simulink model "microgrid_4DER_2019"  (R2019a)
settings: Solver=VariableStepAuto  StartTime=0.0  StopTime=10  RelTol=1e-3
values from neighbouring files (symbols this model uses):
  cf1 = 50 * 1e-6    (= 5e-05)    [parameters.m]
  F1 = 0.75    [parameters.m]
  kic1 = 16e3    (= 16000)    [parameters.m]
  kiv1 = 390    [parameters.m]
  kpc1 = 10.5    [parameters.m]
  kpv1 = 0.05    [parameters.m]
  Lc1 = 0.35 * 1e-3    (= 0.00035)    [parameters.m]
  Lf1 = 1.35 * 1e-3    (= 0.00135)    [parameters.m]
  mp1 = 9.4 * 1e-5    (= 9.4e-05)    [parameters.m]
  nq1 = 1.3 * 1e-3    (= 0.0013)    [parameters.m]
  Rc1 = 0.03    [parameters.m]
  Rf1 = 0.1    [parameters.m]
  Tss = 2.5e-6    (= 2.5e-06)    [parameters.m]
  wb1 = 50 * 2 * pi    (= 314.159265359)    [parameters.m]
  wc1 = 31.41    [parameters.m]
  wcom = 0 * 2 * pi    (= 0)    [parameters.m]
undefined symbols (not defined in the file or in its folder): L11, L12, L13, Lf, R11, R12, R13
libraries: powerlib x46, powerlib_meascontrol x28
(part 1 of 2)
settings Model: Creator=derek  LastModifiedBy=derek

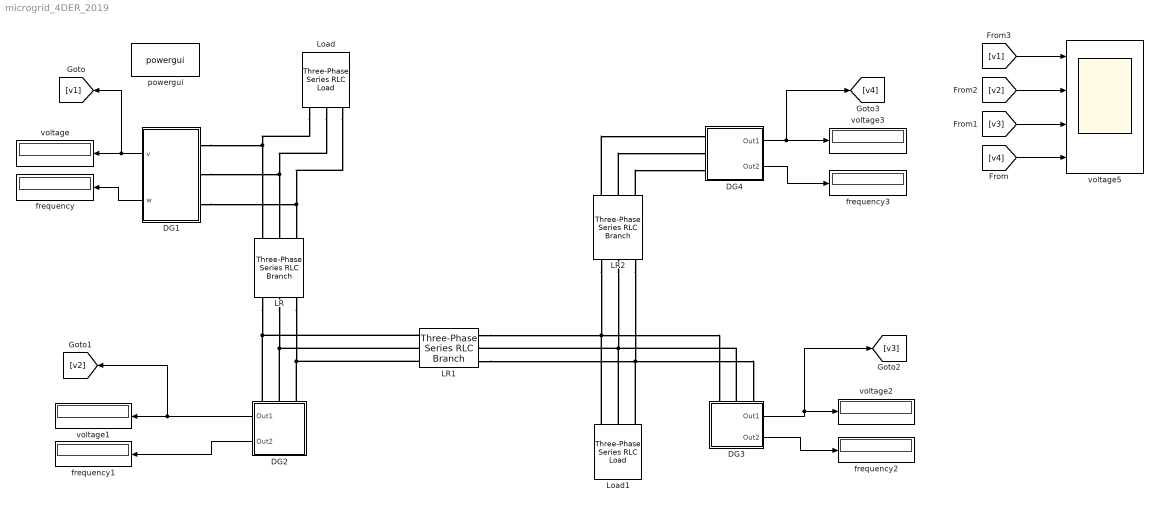
== system microgrid_4DER_2019 ==
  DG1 : Subsystem
  DG2 : Subsystem
      settings: PortSchema="{\"entries\":[{\"content\":{\"sides\":[{\"content\":{\"connectorIds\":[\"LConn1\",\"LConn2\",\"LConn3\"]},\"type\":\"ConnectorPlacement.EquallySpacedRectSide\",\"uuid\":\"9284fba5-743e-4ae1-952f-4876aa99f3ee\"},{\"content\":{\"connectorIds\":[],\"side\":\"RIGHT\"},\"type\":\"ConnectorPlacement.EquallySpacedRectSide\",\"uuid\":\"acb9d5d7-58dc-4066-8a65-0e305600e686\"},{\"content\":{\"connectorIds\":[\"Out1\",\"Out2\"],\"side\":\"TOP\"},\"type\":\"ConnectorPlacement.EquallySpacedRectSide\",\"uuid\":\"239fd259-a6d3-4a4c-98e9-885779a24b56\"}]},\"type\":\"ConnectorPlacement.EquallySpacedConnector\",\"uuid\":\"61a245b7-1af2-4895-a866-301198dca684\"}],\"packageUris\":[\"http://schema.mathworks.com/mf0/Connector/19700101\"],\"version\":\"1.0\"}"
  DG3 : Subsystem
      settings: PortSchema="{\"entries\":[{\"content\":{\"sides\":[{\"content\":{\"connectorIds\":[\"LConn1\",\"LConn2\",\"LConn3\"]},\"type\":\"ConnectorPlacement.EquallySpacedRectSide\",\"uuid\":\"9284fba5-743e-4ae1-952f-4876aa99f3ee\"},{\"content\":{\"connectorIds\":[],\"side\":\"RIGHT\"},\"type\":\"ConnectorPlacement.EquallySpacedRectSide\",\"uuid\":\"acb9d5d7-58dc-4066-8a65-0e305600e686\"},{\"content\":{\"connectorIds\":[],\"side\":\"TOP\"},\"type\":\"ConnectorPlacement.EquallySpacedRectSide\",\"uuid\":\"239fd259-a6d3-4a4c-98e9-885779a24b56\"},{\"content\":{\"connectorIds\":[\"Out1\",\"Out2\"],\"side\":\"BOTTOM\"},\"type\":\"ConnectorPlacement.EquallySpacedRectSide\",\"uuid\":\"f03bd340-3053-4b1f-9b05-34f1428ba472\"}]},\"type\":\"ConnectorPlacement.EquallySpacedConnector\",\"uuid\":\"61a245b7-1af2-4895-a866-301198dca684\"}],\"packageUris\":[\"http://schema.mathworks.com/mf0/Connector/19700101\"],\"version\":\"1.0\"}"
  DG4 : Subsystem
  LR : powerlib/Elements/Three-Phase Series RLC Branch  LConnTagsString=A|B|C  RConnTagsString=A|B|C  BranchType=RL  Resistance=R11  Inductance=L11  Capacitance=Lf  Measurements=None
  LR1 : powerlib/Elements/Three-Phase Series RLC Branch  LConnTagsString=A|B|C  RConnTagsString=A|B|C  BranchType=RL  Resistance=R12  Inductance=L12  Capacitance=Lf  Measurements=None
  LR2 : powerlib/Elements/Three-Phase Series RLC Branch  LConnTagsString=A|B|C  RConnTagsString=A|B|C  BranchType=RL  Resistance=R13  Inductance=L13  Capacitance=Lf  Measurements=None
  Load : powerlib/Elements/Three-Phase Series RLC Load  LConnTagsString=A|B|C  Configuration=Y (grounded)  NominalVoltage=314  Vabc=[1e3 1e3 1e3]  Vabcp=[1e3 1e3 1e3]  NominalFrequency=50  UnbalancedPower=off  ActivePower=12e3  InductivePower=0  CapacitivePower=0  Pabc=[10e3 9e3 11e3]  QLabc=[100 90 110]  QCabc=[100 90 110]  Pabcp=[10e3 9e3 11e3]  QLabcp=[100 90 110]  QCabcp=[100 90 110]  Measurements=None  LoadType=constant Z
  Load1 : powerlib/Elements/Three-Phase Series RLC Load  LConnTagsString=A|B|C  Configuration=Y (grounded)  NominalVoltage=314  Vabc=[1e3 1e3 1e3]  Vabcp=[1e3 1e3 1e3]  NominalFrequency=50  UnbalancedPower=off  ActivePower=15e3  InductivePower=0  CapacitivePower=0  Pabc=[10e3 9e3 11e3]  QLabc=[100 90 110]  QCabc=[100 90 110]  Pabcp=[10e3 9e3 11e3]  QLabcp=[100 90 110]  QCabcp=[100 90 110]  Measurements=None  LoadType=constant Z
  frequency{,1..3} (4 alike) : Display
  powergui : powerlib/powergui  Priority=1  SimulationMode=Discrete  SampleTime=Tss  frequency=60  Iterations=50  frequencyindice=0  Pbase=100e6  ErrMax=1e-4  UnitsV=kV  UnitsW=MW  buscounter=0  FunctionMessages=off  echomessages=off  EnableUseOfTLC=off  CurrentSourceSwitches=off  DisableSnubberDevices=off  DisableRonSwitches=off  DisableVfSwitches=off  DisplayEquations=off  AutomaticDiscreteSolvers=off  SolverType=Tustin/Backward Euler (TBE)  Interpol=off  ExternalGateDelay=off  methode=off  Ts=100  x0status=blocks  SPID=on  SwTol=0  HookPort=off  NonlinearTolerance=0  nMaxIteration=15  ContinueOnMaxIteration=off  RestoreLinks=warning  ResistiveCurrentMeasurement=off  Frange=[0:2:500]  Ylog=off  Xlog=on  ShowGrid=off  save=off  variable=ZData  structure=0  ZoomFFT=off  StartTime=0.0  cycles=1  DisplayStyle=1  fundamental=60  FreqAxis=off  MaxFrequency=1000  frequencyindicesteady=1  RmsSteady=1  display=off
  voltage{,1..3} (4 alike) : Display
  voltage5 : Scope  NumInputPorts=4
  wires:
  DG1/1(v) -> [v1], voltage/1
  DG1/2(w) -> frequency/1
  DG2/1(Out1) -> [v2], voltage1/1
  DG2/2(Out2) -> frequency1/1
  DG4/1(Out1) -> [v4], voltage3/1
  DG4/2(Out2) -> frequency3/1
  DG3/1(Out1) -> [v3], voltage2/1
  DG3/2(Out2) -> frequency2/1
  [v4] -> voltage5/4
  [v3] -> voltage5/3
  [v2] -> voltage5/2
  [v1] -> voltage5/1
  connections:
  DG1/LConn1 -- Load/LConn1 -- LR/LConn1
  DG1/LConn2 -- Load/LConn2 -- LR/LConn2
  DG1/LConn3 -- Load/LConn3 -- LR/LConn3
  LR/RConn1 -- DG2/LConn1 -- LR1/LConn1
  LR/RConn2 -- DG2/LConn2 -- LR1/LConn2
  LR/RConn3 -- DG2/LConn3 -- LR1/LConn3
  LR1/RConn1 -- Load1/LConn1 -- LR2/LConn1 -- DG3/LConn1
  DG3/LConn2 -- LR1/RConn2 -- Load1/LConn2 -- LR2/LConn2
  LR1/RConn3 -- Load1/LConn3 -- LR2/LConn3 -- DG3/LConn3
  LR2/RConn1 -- DG4/LConn1
  LR2/RConn2 -- DG4/LConn2
  LR2/RConn3 -- DG4/LConn3

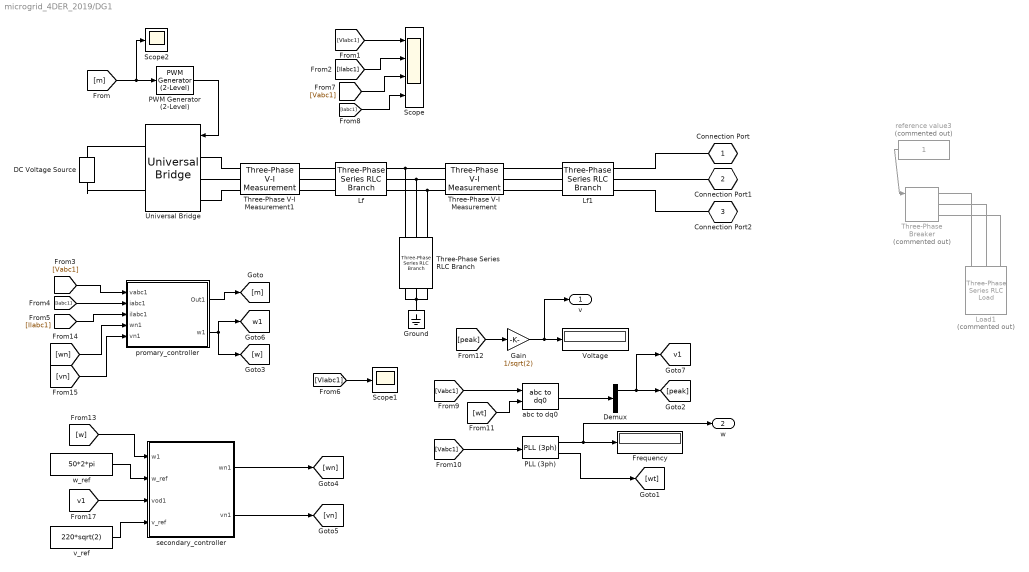
== system microgrid_4DER_2019/DG1 ==
  DC Voltage Source : powerlib/Electrical Sources/DC Voltage Source  Amplitude=600  Measurements=None
  Demux : Demux  Outputs=3
  Frequency : Display
  Gain : Gain  Gain=1/sqrt(2)
  Ground : powerlib/Elements/Ground  LConnTagsString=a
  Lf : powerlib/Elements/Three-Phase Series RLC Branch  LConnTagsString=A|B|C  RConnTagsString=A|B|C  BranchType=RL  Resistance=Rf1  Inductance=Lf1  Capacitance=Lf  Measurements=None
  Lf1 : powerlib/Elements/Three-Phase Series RLC Branch  LConnTagsString=A|B|C  RConnTagsString=A|B|C  BranchType=RL  Resistance=Rc1  Inductance=Lc1  Capacitance=Lf  Measurements=None
  Load1 : powerlib/Elements/Three-Phase Series RLC Load  Commented=on  LConnTagsString=A|B|C  Configuration=Y (grounded)  NominalVoltage=314  Vabc=[1e3 1e3 1e3]  Vabcp=[1e3 1e3 1e3]  NominalFrequency=50  UnbalancedPower=off  ActivePower=20e3  InductivePower=0  CapacitivePower=0  Pabc=[10e3 9e3 11e3]  QLabc=[100 90 110]  QCabc=[100 90 110]  Pabcp=[10e3 9e3 11e3]  QLabcp=[100 90 110]  QCabcp=[100 90 110]  Measurements=None  LoadType=constant Z
  PLL (3ph) : powerlib_meascontrol/PLL/PLL (3ph)  Fmin=45  Par_Init=[0, 50]  ParK=[180, 3200, 1]  TcD=1e-4  MaxRateChangeFreq=12  FilterCutOffFreq=25  Ts=Tss  AGC=on
  PWM Generator (2-Level) : powerlib_meascontrol/Pulse & Signal Generators/PWM Generator (2-Level)  ModulatorType=Three-phase bridge (6 pulses)  ModulatorMode=Unsynchronized  Fc=fsw  Pc=90  nF=27  MinMax="[ -1  1 ]"  SamplingTechnique=Natural  ModulatingSignals=off  m=0.8  Freq=60  Phase=0  Ts=Tss  ShowCarrierOutport=off
  Scope : Scope  NumInputPorts=4
  Scope1 : Scope
  Scope2 : Scope
  Three-Phase Series RLC Branch : powerlib/Elements/Three-Phase Series RLC Branch  LConnTagsString=A|B|C  RConnTagsString=A|B|C  BranchType=RC  Resistance=1e-6  Inductance=1e-3  Capacitance=cf1  Measurements=None
  Three-Phase V-I Measurement : powerlib/Measurements/Three-Phase V-I Measurement  VoltageMeasurement=phase-to-phase  SetLabelV=on  LabelV=Vabc1  Vpu=off  VpuLL=off  CurrentMeasurement=yes  SetLabelI=on  LabelI=Iabc1  Ipu=off  Pbase=100e6  Vbase=500e3  OutputType=Complex  PhasorSimulation=off  PSBequivalent=0
  Three-Phase V-I Measurement1 : powerlib/Measurements/Three-Phase V-I Measurement  VoltageMeasurement=phase-to-phase  SetLabelV=on  LabelV=Vlabc1  Vpu=off  VpuLL=off  CurrentMeasurement=yes  SetLabelI=on  LabelI=Ilabc1  Ipu=off  Pbase=100e6  Vbase=500e3  OutputType=Complex  PhasorSimulation=off  PSBequivalent=0
  Three-Phase Breaker : powerlib/Elements/Three-Phase Breaker  Commented=on  InitialState=open  SwitchA=on  SwitchB=on  SwitchC=on  SwitchTimes="[1/60  5/60]"  External=on  BreakerResistance=0.01  SnubberResistance=1e6  SnubberCapacitance=inf  Measurements=None
  Universal Bridge : powerlib/Power Electronics/Universal Bridge  Arms=3  SnubberResistance=1e5  SnubberCapacitance=inf  Device=IGBT / Diodes  Ron=1e-3  Lon=0  ForwardVoltages="[  0  0  ]"  ForwardVoltage=0  GTOparameters=[ 10e-6 , 20e-6 ]  IGBTparameters=[ 1e-6 , 2e-6 ]  Measurements=None  Measurements_2=None  converterType=Rectifier
  Voltage : Display
  abc to dq0 : powerlib_meascontrol/Transformations/abc to dq0  Alignment=90 degrees behind phase A axis
  promary_controller : Subsystem
  reference value3 : Constant  Commented=on
  secondary_controller : Subsystem
  v_ref : Constant  Value=220*sqrt(2)
  w_ref : Constant  Value=50*2*pi
  Connection Port : PMIOPort  Tag=PMCPort  Side=Left
  Connection Port1 : PMIOPort  Tag=PMCPort  Port=2  Side=Left
  Connection Port2 : PMIOPort  Tag=PMCPort  Port=3  Side=Left
  v : Outport
  w : Outport  Port=2
  tag scope: v1=global, w1=global
  wires:
  [Ilabc1] -> Scope/2
  [Iabc1] -> Scope/4
  [Iabc1] -> promary_controller/2(iabc1)
  [Vlabc1] -> Scope1/1
  [Vlabc1] -> Scope/1
  Gain/1 -> v/1, Voltage/1
  PLL (3ph)/2 -> [wt]
  reference value3/1 -> Three-Phase Breaker/1
  PWM Generator (2-Level)/1 -> Universal Bridge/1
  [Ilabc1] -> promary_controller/3(ilabc1)
  [Vabc1] -> promary_controller/1(vabc1)
  Demux/1 -> [v1], [peak]
  abc to dq0/1 -> Demux/1
  [Vabc1] -> abc to dq0/1
  [Vabc1] -> PLL (3ph)/1
  promary_controller/1(Out1) -> [m]
  [peak] -> Gain/1
  [wt] -> abc to dq0/2
  [m] -> Scope2/1, PWM Generator (2-Level)/1
  PLL (3ph)/1 -> w/1, Frequency/1
  [Vabc1] -> Scope/3
  [w] -> secondary_controller/1(w1)
  promary_controller/2(w1) -> [w1], [w]
  v_ref/1 -> secondary_controller/4(v_ref)
  secondary_controller/1(wn1) -> [wn]
  [wn] -> promary_controller/4(wn1)
  secondary_controller/2(vn1) -> [vn]
  [vn] -> promary_controller/5(vn1)
  [v1] -> secondary_controller/3(vod1)
  w_ref/1 -> secondary_controller/2(w_ref)
  connections:
  Lf1/LConn3 -- Three-Phase V-I Measurement/RConn3
  Three-Phase Breaker/RConn2 -- Load1/LConn2
  Lf1/LConn2 -- Three-Phase V-I Measurement/RConn2
  Connection Port2/RConn1 -- Lf1/RConn3
  Three-Phase Breaker/RConn3 -- Load1/LConn3
  Three-Phase V-I Measurement1/RConn3 -- Lf/LConn3
  Three-Phase V-I Measurement/RConn1 -- Lf1/LConn1
  Three-Phase V-I Measurement1/LConn3 -- Universal Bridge/LConn3
  Three-Phase V-I Measurement1/RConn2 -- Lf/LConn2
  Ground/LConn1 -- Three-Phase Series RLC Branch/RConn3 -- Three-Phase Series RLC Branch/RConn2 -- Three-Phase Series RLC Branch/RConn1
  Lf/RConn2 -- Three-Phase V-I Measurement/LConn2 -- Three-Phase Series RLC Branch/LConn2
  Three-Phase V-I Measurement1/RConn1 -- Lf/LConn1
  Three-Phase V-I Measurement1/LConn2 -- Universal Bridge/LConn2
  Connection Port/RConn1 -- Lf1/RConn1
  DC Voltage Source/RConn1 -- Universal Bridge/RConn1
  Connection Port1/RConn1 -- Lf1/RConn2
  Lf/RConn3 -- Three-Phase V-I Measurement/LConn3 -- Three-Phase Series RLC Branch/LConn3
  Three-Phase Breaker/RConn1 -- Load1/LConn1
  Lf/RConn1 -- Three-Phase V-I Measurement/LConn1 -- Three-Phase Series RLC Branch/LConn1
  DC Voltage Source/LConn1 -- Universal Bridge/RConn2
  Universal Bridge/LConn1 -- Three-Phase V-I Measurement1/LConn1

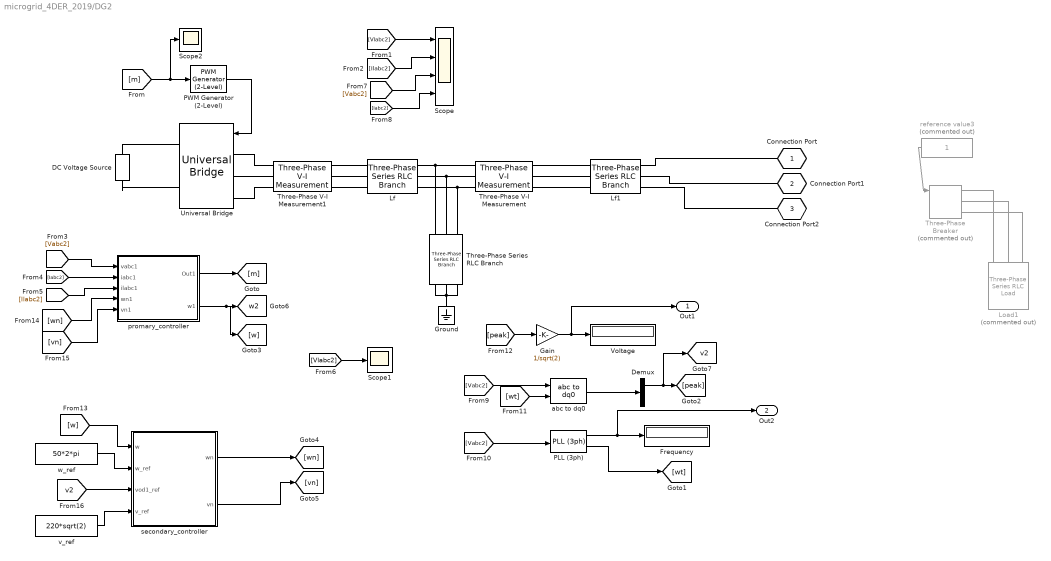
== system microgrid_4DER_2019/DG2 ==
  DC Voltage Source : powerlib/Electrical Sources/DC Voltage Source  Amplitude=600  Measurements=None
  Demux : Demux  Outputs=3
  Frequency : Display
  Gain : Gain  Gain=1/sqrt(2)
  Ground : powerlib/Elements/Ground  LConnTagsString=a
  Lf : powerlib/Elements/Three-Phase Series RLC Branch  LConnTagsString=A|B|C  RConnTagsString=A|B|C  BranchType=RL  Resistance=Rf1  Inductance=Lf1  Capacitance=Lf  Measurements=None
  Lf1 : powerlib/Elements/Three-Phase Series RLC Branch  LConnTagsString=A|B|C  RConnTagsString=A|B|C  BranchType=RL  Resistance=Rc1  Inductance=Lc1  Capacitance=Lf  Measurements=None
  Load1 : powerlib/Elements/Three-Phase Series RLC Load  Commented=on  LConnTagsString=A|B|C  Configuration=Y (grounded)  NominalVoltage=314  Vabc=[1e3 1e3 1e3]  Vabcp=[1e3 1e3 1e3]  NominalFrequency=50  UnbalancedPower=off  ActivePower=20e3  InductivePower=0  CapacitivePower=0  Pabc=[10e3 9e3 11e3]  QLabc=[100 90 110]  QCabc=[100 90 110]  Pabcp=[10e3 9e3 11e3]  QLabcp=[100 90 110]  QCabcp=[100 90 110]  Measurements=None  LoadType=constant Z
  PLL (3ph) : powerlib_meascontrol/PLL/PLL (3ph)  Fmin=45  Par_Init=[0, 50]  ParK=[180, 3200, 1]  TcD=1e-4  MaxRateChangeFreq=12  FilterCutOffFreq=25  Ts=Tss  AGC=on
  PWM Generator (2-Level) : powerlib_meascontrol/Pulse & Signal Generators/PWM Generator (2-Level)  ModulatorType=Three-phase bridge (6 pulses)  ModulatorMode=Unsynchronized  Fc=fsw  Pc=90  nF=27  MinMax="[ -1  1 ]"  SamplingTechnique=Natural  ModulatingSignals=off  m=0.8  Freq=60  Phase=0  Ts=Tss  ShowCarrierOutport=off
  Scope : Scope  NumInputPorts=4
  Scope1 : Scope
  Scope2 : Scope
  Three-Phase Series RLC Branch : powerlib/Elements/Three-Phase Series RLC Branch  LConnTagsString=A|B|C  RConnTagsString=A|B|C  BranchType=RC  Resistance=1e-6  Inductance=1e-3  Capacitance=cf1  Measurements=None
  Three-Phase V-I Measurement : powerlib/Measurements/Three-Phase V-I Measurement  VoltageMeasurement=phase-to-phase  SetLabelV=on  LabelV=Vabc2  Vpu=off  VpuLL=off  CurrentMeasurement=yes  SetLabelI=on  LabelI=Iabc2  Ipu=off  Pbase=100e6  Vbase=500e3  OutputType=Complex  PhasorSimulation=off  PSBequivalent=0
  Three-Phase V-I Measurement1 : powerlib/Measurements/Three-Phase V-I Measurement  VoltageMeasurement=phase-to-phase  SetLabelV=on  LabelV=Vlabc2  Vpu=off  VpuLL=off  CurrentMeasurement=yes  SetLabelI=on  LabelI=Ilabc2  Ipu=off  Pbase=100e6  Vbase=500e3  OutputType=Complex  PhasorSimulation=off  PSBequivalent=0
  Three-Phase Breaker : powerlib/Elements/Three-Phase Breaker  Commented=on  InitialState=open  SwitchA=on  SwitchB=on  SwitchC=on  SwitchTimes="[1/60  5/60]"  External=on  BreakerResistance=0.01  SnubberResistance=1e6  SnubberCapacitance=inf  Measurements=None
  Universal Bridge : powerlib/Power Electronics/Universal Bridge  Arms=3  SnubberResistance=1e5  SnubberCapacitance=inf  Device=IGBT / Diodes  Ron=1e-3  Lon=0  ForwardVoltages="[  0  0  ]"  ForwardVoltage=0  GTOparameters=[ 10e-6 , 20e-6 ]  IGBTparameters=[ 1e-6 , 2e-6 ]  Measurements=None  Measurements_2=None  converterType=Rectifier
  Voltage : Display
  abc to dq0 : powerlib_meascontrol/Transformations/abc to dq0  Alignment=90 degrees behind phase A axis
  promary_controller : Subsystem
  reference value3 : Constant  Commented=on
  secondary_controller : Subsystem
  v_ref : Constant  Value=220*sqrt(2)
  w_ref : Constant  Value=50*2*pi
  Connection Port : PMIOPort  Tag=PMCPort  Side=Left
  Connection Port1 : PMIOPort  Tag=PMCPort  Port=2  Side=Left
  Connection Port2 : PMIOPort  Tag=PMCPort  Port=3  Side=Left
  Out1 : Outport
  Out2 : Outport  Port=2
  tag scope: v2=global, w2=global
  wires:
  [Ilabc2] -> Scope/2
  [Iabc2] -> Scope/4
  [Vlabc2] -> Scope1/1
  [Vlabc2] -> Scope/1
  Gain/1 -> Out1/1, Voltage/1
  PLL (3ph)/2 -> [wt]
  reference value3/1 -> Three-Phase Breaker/1
  PWM Generator (2-Level)/1 -> Universal Bridge/1
  Demux/1 -> [v2], [peak]
  abc to dq0/1 -> Demux/1
  [Vabc2] -> abc to dq0/1
  [Vabc2] -> PLL (3ph)/1
  [peak] -> Gain/1
  [wt] -> abc to dq0/2
  [m] -> Scope2/1, PWM Generator (2-Level)/1
  PLL (3ph)/1 -> Out2/1, Frequency/1
  [Vabc2] -> Scope/3
  [Iabc2] -> promary_controller/2(iabc1)
  [Vabc2] -> promary_controller/1(vabc1)
  [wn] -> promary_controller/4(wn1)
  promary_controller/1(Out1) -> [m]
  promary_controller/2(w1) -> [w], [w2]
  [vn] -> promary_controller/5(vn1)
  [Ilabc2] -> promary_controller/3(ilabc1)
  secondary_controller/2(vn) -> [vn]
  secondary_controller/1(wn) -> [wn]
  [v2] -> secondary_controller/3(vod1_ref)
  w_ref/1 -> secondary_controller/2(w_ref)
  [w] -> secondary_controller/1(w)
  v_ref/1 -> secondary_controller/4(v_ref)
  connections:
  Lf1/LConn3 -- Three-Phase V-I Measurement/RConn3
  Three-Phase Breaker/RConn2 -- Load1/LConn2
  Lf1/LConn2 -- Three-Phase V-I Measurement/RConn2
  Connection Port2/RConn1 -- Lf1/RConn3
  Three-Phase Breaker/RConn3 -- Load1/LConn3
  Three-Phase V-I Measurement1/RConn3 -- Lf/LConn3
  Three-Phase V-I Measurement/RConn1 -- Lf1/LConn1
  Three-Phase V-I Measurement1/LConn3 -- Universal Bridge/LConn3
  Three-Phase V-I Measurement1/RConn2 -- Lf/LConn2
  Ground/LConn1 -- Three-Phase Series RLC Branch/RConn3 -- Three-Phase Series RLC Branch/RConn2 -- Three-Phase Series RLC Branch/RConn1
  Lf/RConn2 -- Three-Phase V-I Measurement/LConn2 -- Three-Phase Series RLC Branch/LConn2
  Three-Phase V-I Measurement1/RConn1 -- Lf/LConn1
  Three-Phase V-I Measurement1/LConn2 -- Universal Bridge/LConn2
  Connection Port/RConn1 -- Lf1/RConn1
  DC Voltage Source/RConn1 -- Universal Bridge/RConn1
  Connection Port1/RConn1 -- Lf1/RConn2
  Lf/RConn3 -- Three-Phase V-I Measurement/LConn3 -- Three-Phase Series RLC Branch/LConn3
  Three-Phase Breaker/RConn1 -- Load1/LConn1
  Lf/RConn1 -- Three-Phase V-I Measurement/LConn1 -- Three-Phase Series RLC Branch/LConn1
  DC Voltage Source/LConn1 -- Universal Bridge/RConn2
  Universal Bridge/LConn1 -- Three-Phase V-I Measurement1/LConn1

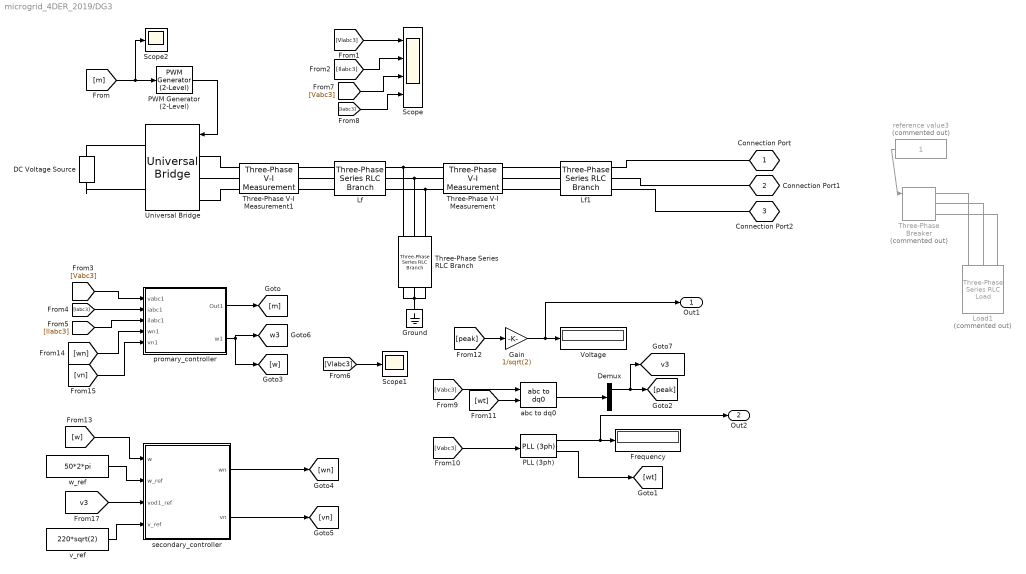
== system microgrid_4DER_2019/DG3 ==
  DC Voltage Source : powerlib/Electrical Sources/DC Voltage Source  Amplitude=600  Measurements=None
  Demux : Demux  Outputs=3
  Frequency : Display
  Gain : Gain  Gain=1/sqrt(2)
  Ground : powerlib/Elements/Ground  LConnTagsString=a
  Lf : powerlib/Elements/Three-Phase Series RLC Branch  LConnTagsString=A|B|C  RConnTagsString=A|B|C  BranchType=RL  Resistance=Rf1  Inductance=Lf1  Capacitance=Lf  Measurements=None
  Lf1 : powerlib/Elements/Three-Phase Series RLC Branch  LConnTagsString=A|B|C  RConnTagsString=A|B|C  BranchType=RL  Resistance=Rc1  Inductance=Lc1  Capacitance=Lf  Measurements=None
  Load1 : powerlib/Elements/Three-Phase Series RLC Load  Commented=on  LConnTagsString=A|B|C  Configuration=Y (grounded)  NominalVoltage=314  Vabc=[1e3 1e3 1e3]  Vabcp=[1e3 1e3 1e3]  NominalFrequency=50  UnbalancedPower=off  ActivePower=20e3  InductivePower=0  CapacitivePower=0  Pabc=[10e3 9e3 11e3]  QLabc=[100 90 110]  QCabc=[100 90 110]  Pabcp=[10e3 9e3 11e3]  QLabcp=[100 90 110]  QCabcp=[100 90 110]  Measurements=None  LoadType=constant Z
  PLL (3ph) : powerlib_meascontrol/PLL/PLL (3ph)  Fmin=45  Par_Init=[0, 50]  ParK=[180, 3200, 1]  TcD=1e-4  MaxRateChangeFreq=12  FilterCutOffFreq=25  Ts=Tss  AGC=on
  PWM Generator (2-Level) : powerlib_meascontrol/Pulse & Signal Generators/PWM Generator (2-Level)  ModulatorType=Three-phase bridge (6 pulses)  ModulatorMode=Unsynchronized  Fc=fsw  Pc=90  nF=27  MinMax="[ -1  1 ]"  SamplingTechnique=Natural  ModulatingSignals=off  m=0.8  Freq=60  Phase=0  Ts=Tss  ShowCarrierOutport=off
  Scope : Scope  NumInputPorts=4
  Scope1 : Scope
  Scope2 : Scope
  Three-Phase Series RLC Branch : powerlib/Elements/Three-Phase Series RLC Branch  LConnTagsString=A|B|C  RConnTagsString=A|B|C  BranchType=RC  Resistance=1e-6  Inductance=1e-3  Capacitance=cf1  Measurements=None
  Three-Phase V-I Measurement : powerlib/Measurements/Three-Phase V-I Measurement  VoltageMeasurement=phase-to-phase  SetLabelV=on  LabelV=Vabc3  Vpu=off  VpuLL=off  CurrentMeasurement=yes  SetLabelI=on  LabelI=Iabc3  Ipu=off  Pbase=100e6  Vbase=500e3  OutputType=Complex  PhasorSimulation=off  PSBequivalent=0
  Three-Phase V-I Measurement1 : powerlib/Measurements/Three-Phase V-I Measurement  VoltageMeasurement=phase-to-phase  SetLabelV=on  LabelV=Vlabc3  Vpu=off  VpuLL=off  CurrentMeasurement=yes  SetLabelI=on  LabelI=Ilabc3  Ipu=off  Pbase=100e6  Vbase=500e3  OutputType=Complex  PhasorSimulation=off  PSBequivalent=0
  Three-Phase Breaker : powerlib/Elements/Three-Phase Breaker  Commented=on  InitialState=open  SwitchA=on  SwitchB=on  SwitchC=on  SwitchTimes="[1/60  5/60]"  External=on  BreakerResistance=0.01  SnubberResistance=1e6  SnubberCapacitance=inf  Measurements=None
  Universal Bridge : powerlib/Power Electronics/Universal Bridge  Arms=3  SnubberResistance=1e5  SnubberCapacitance=inf  Device=IGBT / Diodes  Ron=1e-3  Lon=0  ForwardVoltages="[  0  0  ]"  ForwardVoltage=0  GTOparameters=[ 10e-6 , 20e-6 ]  IGBTparameters=[ 1e-6 , 2e-6 ]  Measurements=None  Measurements_2=None  converterType=Rectifier
  Voltage : Display
  abc to dq0 : powerlib_meascontrol/Transformations/abc to dq0  Alignment=90 degrees behind phase A axis
  promary_controller : Subsystem
  reference value3 : Constant  Commented=on
  secondary_controller : Subsystem
  v_ref : Constant  Value=220*sqrt(2)
  w_ref : Constant  Value=50*2*pi
  Connection Port : PMIOPort  Tag=PMCPort  Side=Left
  Connection Port1 : PMIOPort  Tag=PMCPort  Port=2  Side=Left
  Connection Port2 : PMIOPort  Tag=PMCPort  Port=3  Side=Left
  Out1 : Outport
  Out2 : Outport  Port=2
  tag scope: v3=global, w3=global
  wires:
  [Ilabc3] -> Scope/2
  [Iabc3] -> Scope/4
  [Vlabc3] -> Scope1/1
  [Vlabc3] -> Scope/1
  Gain/1 -> Out1/1, Voltage/1
  PLL (3ph)/2 -> [wt]
  reference value3/1 -> Three-Phase Breaker/1
  PWM Generator (2-Level)/1 -> Universal Bridge/1
  Demux/1 -> [peak], [v3]
  abc to dq0/1 -> Demux/1
  [Vabc3] -> abc to dq0/1
  [Vabc3] -> PLL (3ph)/1
  [peak] -> Gain/1
  [wt] -> abc to dq0/2
  [m] -> Scope2/1, PWM Generator (2-Level)/1
  PLL (3ph)/1 -> Out2/1, Frequency/1
  [Vabc3] -> Scope/3
  [Vabc3] -> promary_controller/1(vabc1)
  [Ilabc3] -> promary_controller/3(ilabc1)
  [wn] -> promary_controller/4(wn1)
  promary_controller/2(w1) -> [w3], [w]
  [Iabc3] -> promary_controller/2(iabc1)
  [vn] -> promary_controller/5(vn1)
  promary_controller/1(Out1) -> [m]
  [v3] -> secondary_controller/3(vod1_ref)
  [w] -> secondary_controller/1(w)
  v_ref/1 -> secondary_controller/4(v_ref)
  w_ref/1 -> secondary_controller/2(w_ref)
  secondary_controller/1(wn) -> [wn]
  secondary_controller/2(vn) -> [vn]
  connections:
  Lf1/LConn3 -- Three-Phase V-I Measurement/RConn3
  Three-Phase Breaker/RConn2 -- Load1/LConn2
  Lf1/LConn2 -- Three-Phase V-I Measurement/RConn2
  Connection Port2/RConn1 -- Lf1/RConn3
  Three-Phase Breaker/RConn3 -- Load1/LConn3
  Three-Phase V-I Measurement1/RConn3 -- Lf/LConn3
  Three-Phase V-I Measurement/RConn1 -- Lf1/LConn1
  Three-Phase V-I Measurement1/LConn3 -- Universal Bridge/LConn3
  Three-Phase V-I Measurement1/RConn2 -- Lf/LConn2
  Ground/LConn1 -- Three-Phase Series RLC Branch/RConn3 -- Three-Phase Series RLC Branch/RConn2 -- Three-Phase Series RLC Branch/RConn1
  Lf/RConn2 -- Three-Phase V-I Measurement/LConn2 -- Three-Phase Series RLC Branch/LConn2
  Three-Phase V-I Measurement1/RConn1 -- Lf/LConn1
  Three-Phase V-I Measurement1/LConn2 -- Universal Bridge/LConn2
  Connection Port/RConn1 -- Lf1/RConn1
  DC Voltage Source/RConn1 -- Universal Bridge/RConn1
  Connection Port1/RConn1 -- Lf1/RConn2
  Lf/RConn3 -- Three-Phase V-I Measurement/LConn3 -- Three-Phase Series RLC Branch/LConn3
  Three-Phase Breaker/RConn1 -- Load1/LConn1
  Lf/RConn1 -- Three-Phase V-I Measurement/LConn1 -- Three-Phase Series RLC Branch/LConn1
  DC Voltage Source/LConn1 -- Universal Bridge/RConn2
  Universal Bridge/LConn1 -- Three-Phase V-I Measurement1/LConn1

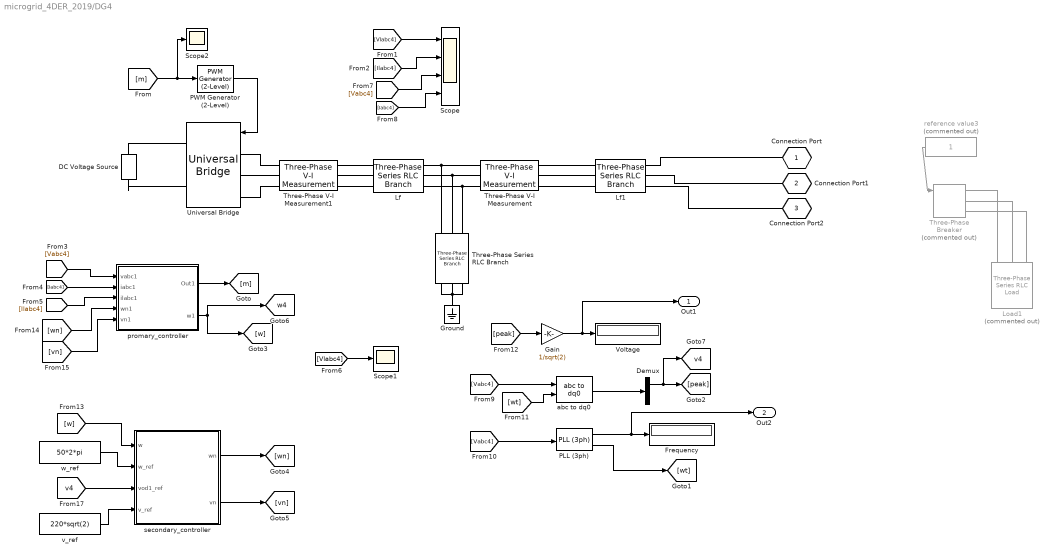
== system microgrid_4DER_2019/DG4 ==
  DC Voltage Source : powerlib/Electrical Sources/DC Voltage Source  Amplitude=600  Measurements=None
  Demux : Demux  Outputs=3
  Frequency : Display
  Gain : Gain  Gain=1/sqrt(2)
  Ground : powerlib/Elements/Ground  LConnTagsString=a
  Lf : powerlib/Elements/Three-Phase Series RLC Branch  LConnTagsString=A|B|C  RConnTagsString=A|B|C  BranchType=RL  Resistance=Rf1  Inductance=Lf1  Capacitance=Lf  Measurements=None
  Lf1 : powerlib/Elements/Three-Phase Series RLC Branch  LConnTagsString=A|B|C  RConnTagsString=A|B|C  BranchType=RL  Resistance=Rc1  Inductance=Lc1  Capacitance=Lf  Measurements=None
  Load1 : powerlib/Elements/Three-Phase Series RLC Load  Commented=on  LConnTagsString=A|B|C  Configuration=Y (grounded)  NominalVoltage=314  Vabc=[1e3 1e3 1e3]  Vabcp=[1e3 1e3 1e3]  NominalFrequency=50  UnbalancedPower=off  ActivePower=20e3  InductivePower=0  CapacitivePower=0  Pabc=[10e3 9e3 11e3]  QLabc=[100 90 110]  QCabc=[100 90 110]  Pabcp=[10e3 9e3 11e3]  QLabcp=[100 90 110]  QCabcp=[100 90 110]  Measurements=None  LoadType=constant Z
  PLL (3ph) : powerlib_meascontrol/PLL/PLL (3ph)  Fmin=45  Par_Init=[0, 50]  ParK=[180, 3200, 1]  TcD=1e-4  MaxRateChangeFreq=12  FilterCutOffFreq=25  Ts=Tss  AGC=on
  PWM Generator (2-Level) : powerlib_meascontrol/Pulse & Signal Generators/PWM Generator (2-Level)  ModulatorType=Three-phase bridge (6 pulses)  ModulatorMode=Unsynchronized  Fc=fsw  Pc=90  nF=27  MinMax="[ -1  1 ]"  SamplingTechnique=Natural  ModulatingSignals=off  m=0.8  Freq=60  Phase=0  Ts=Tss  ShowCarrierOutport=off
  Scope : Scope  NumInputPorts=4
  Scope1 : Scope
  Scope2 : Scope
  Three-Phase Series RLC Branch : powerlib/Elements/Three-Phase Series RLC Branch  LConnTagsString=A|B|C  RConnTagsString=A|B|C  BranchType=RC  Resistance=1e-6  Inductance=1e-3  Capacitance=cf1  Measurements=None
  Three-Phase V-I Measurement : powerlib/Measurements/Three-Phase V-I Measurement  VoltageMeasurement=phase-to-phase  SetLabelV=on  LabelV=Vabc4  Vpu=off  VpuLL=off  CurrentMeasurement=yes  SetLabelI=on  LabelI=Iabc4  Ipu=off  Pbase=100e6  Vbase=500e3  OutputType=Complex  PhasorSimulation=off  PSBequivalent=0
  Three-Phase V-I Measurement1 : powerlib/Measurements/Three-Phase V-I Measurement  VoltageMeasurement=phase-to-phase  SetLabelV=on  LabelV=Vlabc4  Vpu=off  VpuLL=off  CurrentMeasurement=yes  SetLabelI=on  LabelI=Ilabc4  Ipu=off  Pbase=100e6  Vbase=500e3  OutputType=Complex  PhasorSimulation=off  PSBequivalent=0
  Three-Phase Breaker : powerlib/Elements/Three-Phase Breaker  Commented=on  InitialState=open  SwitchA=on  SwitchB=on  SwitchC=on  SwitchTimes="[1/60  5/60]"  External=on  BreakerResistance=0.01  SnubberResistance=1e6  SnubberCapacitance=inf  Measurements=None
  Universal Bridge : powerlib/Power Electronics/Universal Bridge  Arms=3  SnubberResistance=1e5  SnubberCapacitance=inf  Device=IGBT / Diodes  Ron=1e-3  Lon=0  ForwardVoltages="[  0  0  ]"  ForwardVoltage=0  GTOparameters=[ 10e-6 , 20e-6 ]  IGBTparameters=[ 1e-6 , 2e-6 ]  Measurements=None  Measurements_2=None  converterType=Rectifier
  Voltage : Display
  abc to dq0 : powerlib_meascontrol/Transformations/abc to dq0  Alignment=90 degrees behind phase A axis
  promary_controller : Subsystem
  reference value3 : Constant  Commented=on
  secondary_controller : Subsystem
  v_ref : Constant  Value=220*sqrt(2)
  w_ref : Constant  Value=50*2*pi
  Connection Port : PMIOPort  Tag=PMCPort  Side=Left
  Connection Port1 : PMIOPort  Tag=PMCPort  Port=2  Side=Left
  Connection Port2 : PMIOPort  Tag=PMCPort  Port=3  Side=Left
  Out1 : Outport
  Out2 : Outport  Port=2
  tag scope: v4=global, w4=global
  wires:
  [Ilabc4] -> Scope/2
  [Iabc4] -> Scope/4
  [Vlabc4] -> Scope1/1
  [Vlabc4] -> Scope/1
  Gain/1 -> Out1/1, Voltage/1
  PLL (3ph)/2 -> [wt]
  reference value3/1 -> Three-Phase Breaker/1
  PWM Generator (2-Level)/1 -> Universal Bridge/1
  Demux/1 -> [v4], [peak]
  abc to dq0/1 -> Demux/1
  [Vabc4] -> abc to dq0/1
  [Vabc4] -> PLL (3ph)/1
  [peak] -> Gain/1
  [wt] -> abc to dq0/2
  [m] -> Scope2/1, PWM Generator (2-Level)/1
  PLL (3ph)/1 -> Out2/1, Frequency/1
  [Vabc4] -> Scope/3
  [Vabc4] -> promary_controller/1(vabc1)
  [Ilabc4] -> promary_controller/3(ilabc1)
  [wn] -> promary_controller/4(wn1)
  promary_controller/2(w1) -> [w4], [w]
  [Iabc4] -> promary_controller/2(iabc1)
  [vn] -> promary_controller/5(vn1)
  promary_controller/1(Out1) -> [m]
  w_ref/1 -> secondary_controller/2(w_ref)
  v_ref/1 -> secondary_controller/4(v_ref)
  secondary_controller/1(wn) -> [wn]
  secondary_controller/2(vn) -> [vn]
  [w] -> secondary_controller/1(w)
  [v4] -> secondary_controller/3(vod1_ref)
  connections:
  Lf1/LConn3 -- Three-Phase V-I Measurement/RConn3
  Three-Phase Breaker/RConn2 -- Load1/LConn2
  Lf1/LConn2 -- Three-Phase V-I Measurement/RConn2
  Connection Port2/RConn1 -- Lf1/RConn3
  Three-Phase Breaker/RConn3 -- Load1/LConn3
  Three-Phase V-I Measurement1/RConn3 -- Lf/LConn3
  Three-Phase V-I Measurement/RConn1 -- Lf1/LConn1
  Three-Phase V-I Measurement1/LConn3 -- Universal Bridge/LConn3
  Three-Phase V-I Measurement1/RConn2 -- Lf/LConn2
  Ground/LConn1 -- Three-Phase Series RLC Branch/RConn3 -- Three-Phase Series RLC Branch/RConn2 -- Three-Phase Series RLC Branch/RConn1
  Lf/RConn2 -- Three-Phase V-I Measurement/LConn2 -- Three-Phase Series RLC Branch/LConn2
  Three-Phase V-I Measurement1/RConn1 -- Lf/LConn1
  Three-Phase V-I Measurement1/LConn2 -- Universal Bridge/LConn2
  Connection Port/RConn1 -- Lf1/RConn1
  DC Voltage Source/RConn1 -- Universal Bridge/RConn1
  Connection Port1/RConn1 -- Lf1/RConn2
  Lf/RConn3 -- Three-Phase V-I Measurement/LConn3 -- Three-Phase Series RLC Branch/LConn3
  Three-Phase Breaker/RConn1 -- Load1/LConn1
  Lf/RConn1 -- Three-Phase V-I Measurement/LConn1 -- Three-Phase Series RLC Branch/LConn1
  DC Voltage Source/LConn1 -- Universal Bridge/RConn2
  Universal Bridge/LConn1 -- Three-Phase V-I Measurement1/LConn1

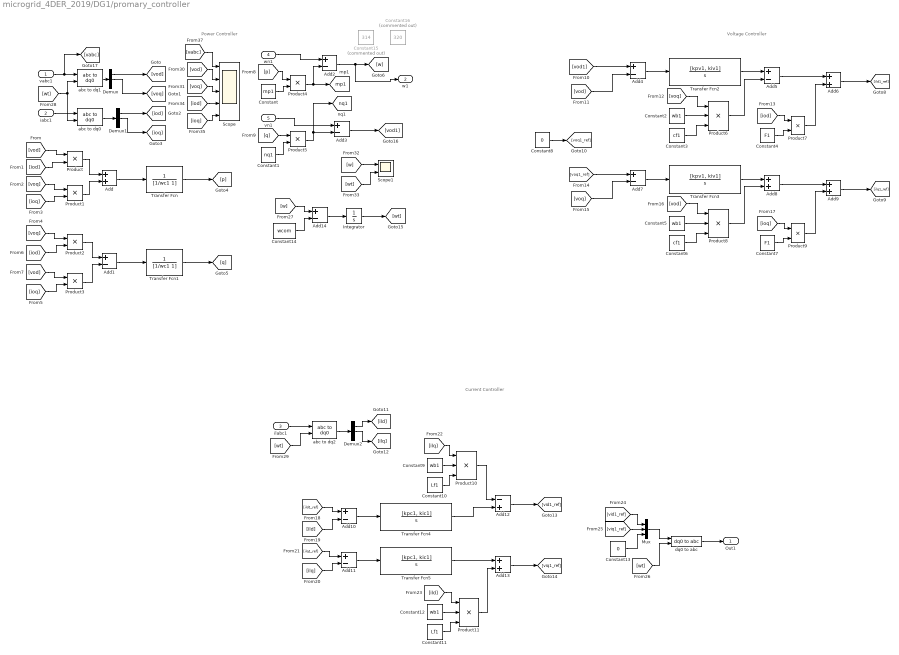
== system microgrid_4DER_2019/DG1/promary_controller ==
  note: Voltage Controller
  note: Power Controller
  note: Current Controller
  vabc1 : Inport
  iabc1 : Inport  Port=2
  ilabc1 : Inport  Port=3
  wn1 : Inport  Port=4
  vn1 : Inport  Port=5
  Add{,6,8..9,13} (5 alike) : Sum
  Add{1..5,7,10..11,14} (9 alike) : Sum  Inputs=+-
  Add12 : Sum  Inputs=-+
  Constant : Constant  Value=mp1
  Constant1 : Constant  Value=nq1
  Constant10 : Constant  Value=Lf1
  Constant11 : Constant  Value=Lf1
  Constant{2,5,9,12} (4 alike) : Constant  Value=wb1
  Constant13 : Constant  Value=0
  Constant14 : Constant  Value=wcom  SampleTime=Tss
  Constant15 : Constant  Commented=on  Value=314
  Constant16 : Constant  Commented=on  Value=320
  Constant3 : Constant  Value=cf1
  Constant4 : Constant  Value=F1
  Constant6 : Constant  Value=cf1
  Constant7 : Constant  Value=F1
  Constant8 : Constant  Value=0
  Demux : Demux  Outputs=3
  Demux1 : Demux  Outputs=3
  Demux2 : Demux  Outputs=3
  Integrator : Integrator
  Mux : Mux  Inputs=3
  Product{,1..5,7,9} (8 alike) : Product
  Product{6,8,10..11} (4 alike) : Product  Inputs=3
  Scope : Scope  NumInputPorts=5
  Scope1 : Scope  NumInputPorts=2
  Transfer Fcn : TransferFcn  Denominator=[1/wc1 1]
  Transfer Fcn1 : TransferFcn  Denominator=[1/wc1 1]
  Transfer Fcn2 : TransferFcn  Numerator=[kpv1, kiv1]  Denominator=[1, 0]
  Transfer Fcn3 : TransferFcn  Numerator=[kpv1, kiv1]  Denominator=[1, 0]
  Transfer Fcn4 : TransferFcn  Numerator=[kpc1, kic1]  Denominator=[1, 0]
  Transfer Fcn5 : TransferFcn  Numerator=[kpc1, kic1]  Denominator=[1, 0]
  abc to dq0 : powerlib_meascontrol/Transformations/abc to dq0  Alignment=90 degrees behind phase A axis
  abc to dq1 : powerlib_meascontrol/Transformations/abc to dq0  Alignment=90 degrees behind phase A axis
  abc to dq2 : powerlib_meascontrol/Transformations/abc to dq0  Alignment=90 degrees behind phase A axis
  dq0 to abc : powerlib_meascontrol/Transformations/dq0 to abc  Alignment=90 degrees behind phase A axis
  Out1 : Outport
  w1 : Outport  Port=2
  tag scope: mp1=global, nq1=global
  wires:
  vabc1/1 -> [vabc], abc to dq1/1
  iabc1/1 -> abc to dq0/1
  Demux/1 -> [vod]
  Demux/2 -> [voq]
  abc to dq1/1 -> Demux/1
  Demux1/2 -> [ioq]
  Demux1/1 -> [iod]
  abc to dq0/1 -> Demux1/1
  [vod] -> Product/1
  [iod] -> Product/2
  [voq] -> Product1/1
  [ioq] -> Product1/2
  Product/1 -> Add/1
  Product1/1 -> Add/2
  Add/1 -> Transfer Fcn/1
  Transfer Fcn/1 -> [p]
  [voq] -> Product2/1
  [iod] -> Product2/2
  [vod] -> Product3/1
  [ioq] -> Product3/2
  Product2/1 -> Add1/1
  Product3/1 -> Add1/2
  Transfer Fcn1/1 -> [q]
  Add1/1 -> Transfer Fcn1/1
  [p] -> Product4/1
  Constant/1 -> Product4/2
  Product4/1 -> Add2/2, [mp1]
  Add2/1 -> w1/1, [w]
  [q] -> Product5/1
  Constant1/1 -> Product5/2
  Product5/1 -> [nq1], Add3/2
  [vod1] -> Add4/1
  [vod] -> Add4/2
  Add4/1 -> Transfer Fcn2/1
  Transfer Fcn2/1 -> Add5/1
  Constant2/1 -> Product6/2
  [voq] -> Product6/1
  Constant3/1 -> Product6/3
  Product6/1 -> Add5/2
  Add5/1 -> Add6/1
  [iod] -> Product7/1
  Constant4/1 -> Product7/2
  Product7/1 -> Add6/2
  Add6/1 -> [ild1_ref]
  Product8/1 -> Add8/2
  Constant6/1 -> Product8/3
  Add9/1 -> [ilq1_ref]
  Constant7/1 -> Product9/2
  Product9/1 -> Add9/2
  [ioq] -> Product9/1
  Constant5/1 -> Product8/2
  [voq] -> Add7/2
  [voq1_ref] -> Add7/1
  Add7/1 -> Transfer Fcn3/1
  Add8/1 -> Add9/1
  Transfer Fcn3/1 -> Add8/1
  [vod] -> Product8/1
  Constant8/1 -> [voq1_ref]
  ilabc1/1 -> abc to dq2/1
  abc to dq2/1 -> Demux2/1
  Demux2/1 -> [ild]
  Demux2/2 -> [ilq]
  [ild1_ref] -> Add10/1
  [ild] -> Add10/2
  [ilq] -> Add11/2
  [ilq1_ref] -> Add11/1
  Add10/1 -> Transfer Fcn4/1
  Add11/1 -> Transfer Fcn5/1
  Transfer Fcn4/1 -> Add12/2
  [ilq] -> Product10/1
  Constant9/1 -> Product10/2
  Constant10/1 -> Product10/3
  Product10/1 -> Add12/1
  Add12/1 -> [vid1_ref]
  Constant12/1 -> Product11/2
  [ild] -> Product11/1
  Constant11/1 -> Product11/3
  Product11/1 -> Add13/2
  Transfer Fcn5/1 -> Add13/1
  Add13/1 -> [viq1_ref]
  [vid1_ref] -> Mux/1
  [viq1_ref] -> Mux/2
  Mux/1 -> dq0 to abc/1
  dq0 to abc/1 -> Out1/1
  [wt] -> dq0 to abc/2
  Constant13/1 -> Mux/3
  Constant14/1 -> Add14/2
  Add14/1 -> Integrator/1
  Integrator/1 -> [wt]
  [wt] -> abc to dq0/2, abc to dq1/2
  [wt] -> abc to dq2/2
  [w] -> Scope1/1
  [wt] -> Scope1/2
  [ioq] -> Scope/5
  [iod] -> Scope/4
  [voq] -> Scope/3
  [vod] -> Scope/2
  [vabc] -> Scope/1
  [w] -> Add14/1
  vn1/1 -> Add3/1
  wn1/1 -> Add2/1
  Add3/1 -> [vod1]

== system microgrid_4DER_2019/DG1/secondary_controller ==
  w1 : Inport
  w_ref : Inport  Port=2
  vod1 : Inport  Port=3
  v_ref : Inport  Port=4
  Add{1,3,5..6,15..16} (6 alike) : Sum  Inputs=+-
  Add2 : Sum  Inputs=+++
  Add4 : Sum  Inputs=+++
  Gain1 : Gain  Gain=-30
  Gain2 : Gain  Gain=-30
  Integrator1 : Integrator  InitialCondition=50*2*pi
  Integrator2 : Integrator  InitialCondition=220*sqrt(2)
  wn1 : Outport
  vn1 : Outport  Port=2
  wires:
  w1/1 -> Add1/1, Add15/1
  vod1/1 -> Add16/1, Add3/1
  v_ref/1 -> Add16/2
  Integrator1/1 -> wn1/1
  Gain2/1 -> Integrator2/1
  Gain1/1 -> Integrator1/1
  w_ref/1 -> Add15/2
  Integrator2/1 -> vn1/1
  [w2] -> Add1/2
  Add15/1 -> Add2/1
  Add1/1 -> Add2/2
  Add2/1 -> Gain1/1
  [v2] -> Add3/2
  Add16/1 -> Add4/1
  Add3/1 -> Add4/2
  Add4/1 -> Gain2/1
  [mp2] -> Add6/2
  [mp1] -> Add6/1
  Add6/1 -> Add2/3
  [nq2] -> Add5/2
  Add5/1 -> Add4/3
  [nq1] -> Add5/1

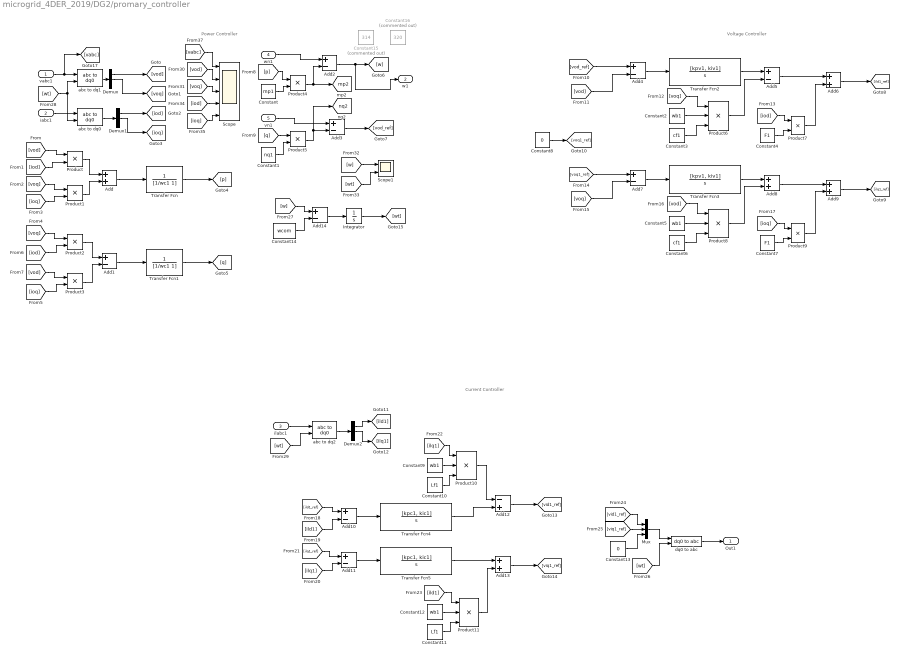
== system microgrid_4DER_2019/DG2/promary_controller ==
  note: Voltage Controller
  note: Power Controller
  note: Current Controller
  vabc1 : Inport
  iabc1 : Inport  Port=2
  ilabc1 : Inport  Port=3
  wn1 : Inport  Port=4
  vn1 : Inport  Port=5
  Add{,6,8..9,13} (5 alike) : Sum
  Add{1..5,7,10..11,14} (9 alike) : Sum  Inputs=+-
  Add12 : Sum  Inputs=-+
  Constant : Constant  Value=mp1
  Constant1 : Constant  Value=nq1
  Constant10 : Constant  Value=Lf1
  Constant11 : Constant  Value=Lf1
  Constant{2,5,9,12} (4 alike) : Constant  Value=wb1
  Constant13 : Constant  Value=0
  Constant14 : Constant  Value=wcom  SampleTime=Tss
  Constant15 : Constant  Commented=on  Value=314
  Constant16 : Constant  Commented=on  Value=320
  Constant3 : Constant  Value=cf1
  Constant4 : Constant  Value=F1
  Constant6 : Constant  Value=cf1
  Constant7 : Constant  Value=F1
  Constant8 : Constant  Value=0
  Demux : Demux  Outputs=3
  Demux1 : Demux  Outputs=3
  Demux2 : Demux  Outputs=3
  Integrator : Integrator
  Mux : Mux  Inputs=3
  Product{,1..5,7,9} (8 alike) : Product
  Product{6,8,10..11} (4 alike) : Product  Inputs=3
  Scope : Scope  NumInputPorts=5
  Scope1 : Scope  NumInputPorts=2
  Transfer Fcn : TransferFcn  Denominator=[1/wc1 1]
  Transfer Fcn1 : TransferFcn  Denominator=[1/wc1 1]
  Transfer Fcn2 : TransferFcn  Numerator=[kpv1, kiv1]  Denominator=[1, 0]
  Transfer Fcn3 : TransferFcn  Numerator=[kpv1, kiv1]  Denominator=[1, 0]
  Transfer Fcn4 : TransferFcn  Numerator=[kpc1, kic1]  Denominator=[1, 0]
  Transfer Fcn5 : TransferFcn  Numerator=[kpc1, kic1]  Denominator=[1, 0]
  abc to dq0 : powerlib_meascontrol/Transformations/abc to dq0  Alignment=90 degrees behind phase A axis
  abc to dq1 : powerlib_meascontrol/Transformations/abc to dq0  Alignment=90 degrees behind phase A axis
  abc to dq2 : powerlib_meascontrol/Transformations/abc to dq0  Alignment=90 degrees behind phase A axis
  dq0 to abc : powerlib_meascontrol/Transformations/dq0 to abc  Alignment=90 degrees behind phase A axis
  Out1 : Outport
  w1 : Outport  Port=2
  tag scope: mp2=global, nq2=global
  wires:
  vabc1/1 -> [vabc], abc to dq1/1
  iabc1/1 -> abc to dq0/1
  Demux/1 -> [vod]
  Demux/2 -> [voq]
  abc to dq1/1 -> Demux/1
  Demux1/2 -> [ioq]
  Demux1/1 -> [iod]
  abc to dq0/1 -> Demux1/1
  [vod] -> Product/1
  [iod] -> Product/2
  [voq] -> Product1/1
  [ioq] -> Product1/2
  Product/1 -> Add/1
  Product1/1 -> Add/2
  Add/1 -> Transfer Fcn/1
  Transfer Fcn/1 -> [p]
  [voq] -> Product2/1
  [iod] -> Product2/2
  [vod] -> Product3/1
  [ioq] -> Product3/2
  Product2/1 -> Add1/1
  Product3/1 -> Add1/2
  Transfer Fcn1/1 -> [q]
  Add1/1 -> Transfer Fcn1/1
  [p] -> Product4/1
  Constant/1 -> Product4/2
  Product4/1 -> [mp2], Add2/2
  Add2/1 -> w1/1, [w]
  [q] -> Product5/1
  Constant1/1 -> Product5/2
  Product5/1 -> [nq2], Add3/2
  Add3/1 -> [vod_ref]
  [vod_ref] -> Add4/1
  [vod] -> Add4/2
  Add4/1 -> Transfer Fcn2/1
  Transfer Fcn2/1 -> Add5/1
  Constant2/1 -> Product6/2
  [voq] -> Product6/1
  Constant3/1 -> Product6/3
  Product6/1 -> Add5/2
  Add5/1 -> Add6/1
  [iod] -> Product7/1
  Constant4/1 -> Product7/2
  Product7/1 -> Add6/2
  Add6/1 -> [ild1_ref]
  Product8/1 -> Add8/2
  Constant6/1 -> Product8/3
  Add9/1 -> [ilq1_ref]
  Constant7/1 -> Product9/2
  Product9/1 -> Add9/2
  [ioq] -> Product9/1
  Constant5/1 -> Product8/2
  [voq] -> Add7/2
  [voq1_ref] -> Add7/1
  Add7/1 -> Transfer Fcn3/1
  Add8/1 -> Add9/1
  Transfer Fcn3/1 -> Add8/1
  [vod] -> Product8/1
  Constant8/1 -> [voq1_ref]
  ilabc1/1 -> abc to dq2/1
  abc to dq2/1 -> Demux2/1
  Demux2/1 -> [ild1]
  Demux2/2 -> [ilq1]
  [ild1_ref] -> Add10/1
  [ild1] -> Add10/2
  [ilq1] -> Add11/2
  [ilq1_ref] -> Add11/1
  Add10/1 -> Transfer Fcn4/1
  Add11/1 -> Transfer Fcn5/1
  Transfer Fcn4/1 -> Add12/2
  [ilq1] -> Product10/1
  Constant9/1 -> Product10/2
  Constant10/1 -> Product10/3
  Product10/1 -> Add12/1
  Add12/1 -> [vid1_ref]
  Constant12/1 -> Product11/2
  [ild1] -> Product11/1
  Constant11/1 -> Product11/3
  Product11/1 -> Add13/2
  Transfer Fcn5/1 -> Add13/1
  Add13/1 -> [viq1_ref]
  [vid1_ref] -> Mux/1
  [viq1_ref] -> Mux/2
  Mux/1 -> dq0 to abc/1
  dq0 to abc/1 -> Out1/1
  [wt] -> dq0 to abc/2
  Constant13/1 -> Mux/3
  Constant14/1 -> Add14/2
  Add14/1 -> Integrator/1
  Integrator/1 -> [wt]
  [wt] -> abc to dq0/2, abc to dq1/2
  [wt] -> abc to dq2/2
  [w] -> Scope1/1
  [wt] -> Scope1/2
  [ioq] -> Scope/5
  [iod] -> Scope/4
  [voq] -> Scope/3
  [vod] -> Scope/2
  [vabc] -> Scope/1
  [w] -> Add14/1
  vn1/1 -> Add3/1
  wn1/1 -> Add2/1

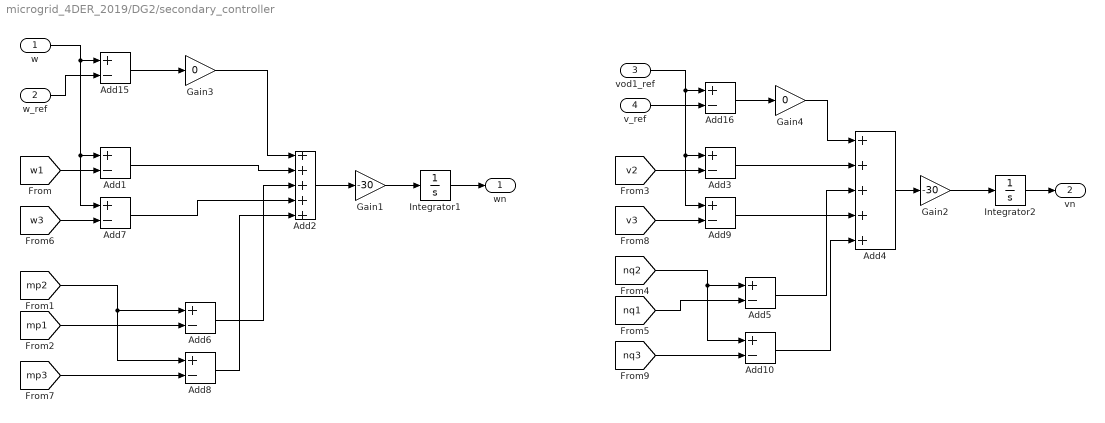
== system microgrid_4DER_2019/DG2/secondary_controller ==
  w : Inport
  w_ref : Inport  Port=2
  vod1_ref : Inport  Port=3
  v_ref : Inport  Port=4
  Add{1,3,5..10,15..16} (10 alike) : Sum  Inputs=+-
  Add2 : Sum  Inputs=+++++
  Add4 : Sum  Inputs=+++++
  Gain1 : Gain  Gain=-30
  Gain2 : Gain  Gain=-30
  Gain3 : Gain  Gain=0
  Gain4 : Gain  Gain=0
  Integrator1 : Integrator  InitialCondition=50*2*pi
  Integrator2 : Integrator  InitialCondition=220*sqrt(2)
  wn : Outport
  vn : Outport  Port=2
  wires:
  w/1 -> Add7/1, Add1/1, Add15/1
  vod1_ref/1 -> Add9/1, Add3/1, Add16/1
  v_ref/1 -> Add16/2
  Integrator1/1 -> wn/1
  Gain2/1 -> Integrator2/1
  Gain1/1 -> Integrator1/1
  w_ref/1 -> Add15/2
  Integrator2/1 -> vn/1
  [w1] -> Add1/2
  Add15/1 -> Gain3/1
  Add1/1 -> Add2/2
  Add2/1 -> Gain1/1
  [v2] -> Add3/2
  Add16/1 -> Gain4/1
  Add3/1 -> Add4/2
  Add4/1 -> Gain2/1
  [mp1] -> Add6/2
  [mp2] -> Add8/1, Add6/1
  Add6/1 -> Add2/3
  [nq1] -> Add5/2
  Add5/1 -> Add4/3
  [nq2] -> Add10/1, Add5/1
  Gain3/1 -> Add2/1
  [w3] -> Add7/2
  [mp3] -> Add8/2
  Gain4/1 -> Add4/1
  [v3] -> Add9/2
  [nq3] -> Add10/2
  Add7/1 -> Add2/4
  Add8/1 -> Add2/5
  Add9/1 -> Add4/4
  Add10/1 -> Add4/5

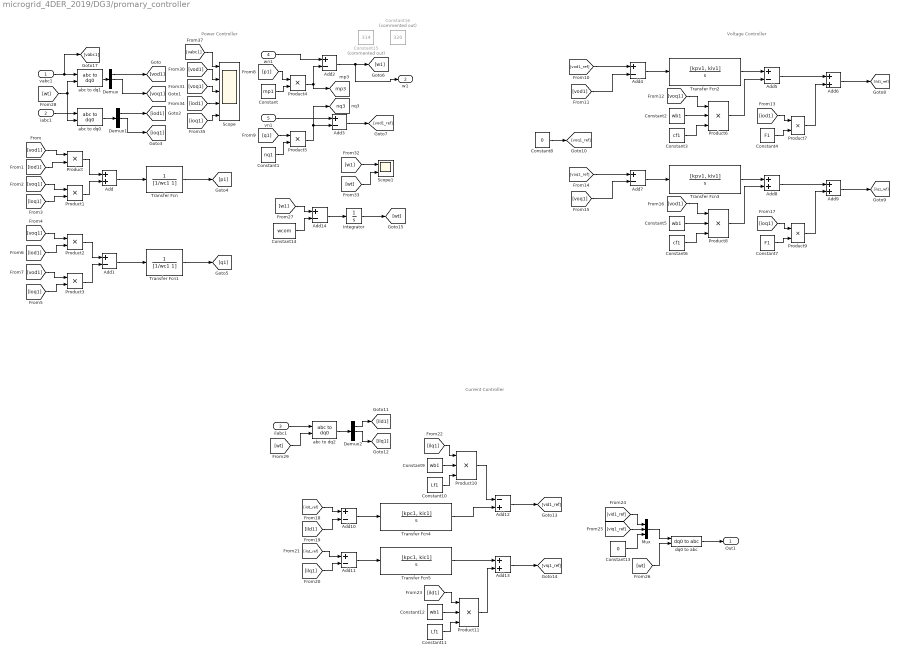
== system microgrid_4DER_2019/DG3/promary_controller ==
  note: Voltage Controller
  note: Power Controller
  note: Current Controller
  vabc1 : Inport
  iabc1 : Inport  Port=2
  ilabc1 : Inport  Port=3
  wn1 : Inport  Port=4
  vn1 : Inport  Port=5
  Add{,6,8..9,13} (5 alike) : Sum
  Add{1..5,7,10..11,14} (9 alike) : Sum  Inputs=+-
  Add12 : Sum  Inputs=-+
  Constant : Constant  Value=mp1
  Constant1 : Constant  Value=nq1
  Constant10 : Constant  Value=Lf1
  Constant11 : Constant  Value=Lf1
  Constant{2,5,9,12} (4 alike) : Constant  Value=wb1
  Constant13 : Constant  Value=0
  Constant14 : Constant  Value=wcom  SampleTime=Tss
  Constant15 : Constant  Commented=on  Value=314
  Constant16 : Constant  Commented=on  Value=320
  Constant3 : Constant  Value=cf1
  Constant4 : Constant  Value=F1
  Constant6 : Constant  Value=cf1
  Constant7 : Constant  Value=F1
  Constant8 : Constant  Value=0
  Demux : Demux  Outputs=3
  Demux1 : Demux  Outputs=3
  Demux2 : Demux  Outputs=3
  Integrator : Integrator
  Mux : Mux  Inputs=3
  Product{,1..5,7,9} (8 alike) : Product
  Product{6,8,10..11} (4 alike) : Product  Inputs=3
  Scope : Scope  NumInputPorts=5
  Scope1 : Scope  NumInputPorts=2
  Transfer Fcn : TransferFcn  Denominator=[1/wc1 1]
  Transfer Fcn1 : TransferFcn  Denominator=[1/wc1 1]
  Transfer Fcn2 : TransferFcn  Numerator=[kpv1, kiv1]  Denominator=[1, 0]
  Transfer Fcn3 : TransferFcn  Numerator=[kpv1, kiv1]  Denominator=[1, 0]
  Transfer Fcn4 : TransferFcn  Numerator=[kpc1, kic1]  Denominator=[1, 0]
  Transfer Fcn5 : TransferFcn  Numerator=[kpc1, kic1]  Denominator=[1, 0]
  abc to dq0 : powerlib_meascontrol/Transformations/abc to dq0  Alignment=90 degrees behind phase A axis
  abc to dq1 : powerlib_meascontrol/Transformations/abc to dq0  Alignment=90 degrees behind phase A axis
  abc to dq2 : powerlib_meascontrol/Transformations/abc to dq0  Alignment=90 degrees behind phase A axis
  dq0 to abc : powerlib_meascontrol/Transformations/dq0 to abc  Alignment=90 degrees behind phase A axis
  Out1 : Outport
  w1 : Outport  Port=2
  tag scope: mp3=global, nq3=global
  wires:
  vabc1/1 -> [vabc1], abc to dq1/1
  iabc1/1 -> abc to dq0/1
  Demux/1 -> [vod1]
  Demux/2 -> [voq1]
  abc to dq1/1 -> Demux/1
  Demux1/2 -> [ioq1]
  Demux1/1 -> [iod1]
  abc to dq0/1 -> Demux1/1
  [vod1] -> Product/1
  [iod1] -> Product/2
  [voq1] -> Product1/1
  [ioq1] -> Product1/2
  Product/1 -> Add/1
  Product1/1 -> Add/2
  Add/1 -> Transfer Fcn/1
  Transfer Fcn/1 -> [p1]
  [voq1] -> Product2/1
  [iod1] -> Product2/2
  [vod1] -> Product3/1
  [ioq1] -> Product3/2
  Product2/1 -> Add1/1
  Product3/1 -> Add1/2
  Transfer Fcn1/1 -> [q1]
  Add1/1 -> Transfer Fcn1/1
  [p1] -> Product4/1
  Constant/1 -> Product4/2
  Product4/1 -> [mp3], Add2/2
  Add2/1 -> w1/1, [w1]
  [q1] -> Product5/1
  Constant1/1 -> Product5/2
  Product5/1 -> [nq3], Add3/2
  Add3/1 -> [vod1_ref]
  [vod1_ref] -> Add4/1
  [vod1] -> Add4/2
  Add4/1 -> Transfer Fcn2/1
  Transfer Fcn2/1 -> Add5/1
  Constant2/1 -> Product6/2
  [voq1] -> Product6/1
  Constant3/1 -> Product6/3
  Product6/1 -> Add5/2
  Add5/1 -> Add6/1
  [iod1] -> Product7/1
  Constant4/1 -> Product7/2
  Product7/1 -> Add6/2
  Add6/1 -> [ild1_ref]
  Product8/1 -> Add8/2
  Constant6/1 -> Product8/3
  Add9/1 -> [ilq1_ref]
  Constant7/1 -> Product9/2
  Product9/1 -> Add9/2
  [ioq1] -> Product9/1
  Constant5/1 -> Product8/2
  [voq1] -> Add7/2
  [voq1_ref] -> Add7/1
  Add7/1 -> Transfer Fcn3/1
  Add8/1 -> Add9/1
  Transfer Fcn3/1 -> Add8/1
  [vod1] -> Product8/1
  Constant8/1 -> [voq1_ref]
  ilabc1/1 -> abc to dq2/1
  abc to dq2/1 -> Demux2/1
  Demux2/1 -> [ild1]
  Demux2/2 -> [ilq1]
  [ild1_ref] -> Add10/1
  [ild1] -> Add10/2
  [ilq1] -> Add11/2
  [ilq1_ref] -> Add11/1
  Add10/1 -> Transfer Fcn4/1
  Add11/1 -> Transfer Fcn5/1
  Transfer Fcn4/1 -> Add12/2
  [ilq1] -> Product10/1
  Constant9/1 -> Product10/2
  Constant10/1 -> Product10/3
  Product10/1 -> Add12/1
  Add12/1 -> [vid1_ref]
  Constant12/1 -> Product11/2
  [ild1] -> Product11/1
  Constant11/1 -> Product11/3
  Product11/1 -> Add13/2
  Transfer Fcn5/1 -> Add13/1
  Add13/1 -> [viq1_ref]
  [vid1_ref] -> Mux/1
  [viq1_ref] -> Mux/2
  Mux/1 -> dq0 to abc/1
  dq0 to abc/1 -> Out1/1
  [wt] -> dq0 to abc/2
  Constant13/1 -> Mux/3
  Constant14/1 -> Add14/2
  Add14/1 -> Integrator/1
  Integrator/1 -> [wt]
  [wt] -> abc to dq0/2, abc to dq1/2
  [wt] -> abc to dq2/2
  [w1] -> Scope1/1
  [wt] -> Scope1/2
  [ioq1] -> Scope/5
  [iod1] -> Scope/4
  [voq1] -> Scope/3
  [vod1] -> Scope/2
  [vabc1] -> Scope/1
  [w1] -> Add14/1
  vn1/1 -> Add3/1
  wn1/1 -> Add2/1

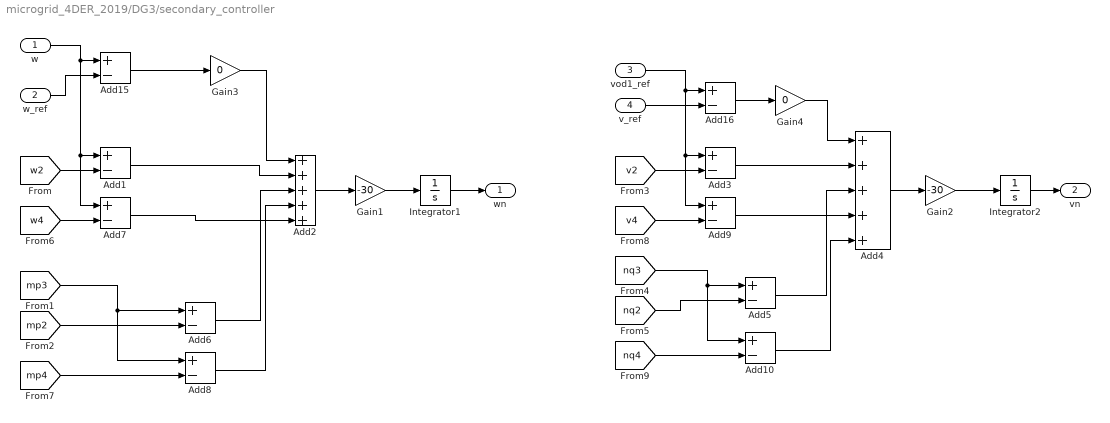
== system microgrid_4DER_2019/DG3/secondary_controller ==
  w : Inport
  w_ref : Inport  Port=2
  vod1_ref : Inport  Port=3
  v_ref : Inport  Port=4
  Add{1,3,5..10,15..16} (10 alike) : Sum  Inputs=+-
  Add2 : Sum  Inputs=+++++
  Add4 : Sum  Inputs=+++++
  Gain1 : Gain  Gain=-30
  Gain2 : Gain  Gain=-30
  Gain3 : Gain  Gain=0
  Gain4 : Gain  Gain=0
  Integrator1 : Integrator  InitialCondition=50*2*pi
  Integrator2 : Integrator  InitialCondition=220*sqrt(2)
  wn : Outport
  vn : Outport  Port=2
  wires:
  w/1 -> Add7/1, Add1/1, Add15/1
  vod1_ref/1 -> Add9/1, Add3/1, Add16/1
  v_ref/1 -> Add16/2
  Integrator1/1 -> wn/1
  Gain2/1 -> Integrator2/1
  Gain1/1 -> Integrator1/1
  w_ref/1 -> Add15/2
  Integrator2/1 -> vn/1
  [w2] -> Add1/2
  Add15/1 -> Gain3/1
  Add1/1 -> Add2/2
  Add2/1 -> Gain1/1
  [v2] -> Add3/2
  Add16/1 -> Gain4/1
  Add3/1 -> Add4/2
  Add4/1 -> Gain2/1
  [mp2] -> Add6/2
  [mp3] -> Add8/1, Add6/1
  Add6/1 -> Add2/3
  [nq2] -> Add5/2
  Add5/1 -> Add4/3
  [nq3] -> Add10/1, Add5/1
  Gain3/1 -> Add2/1
  [w4] -> Add7/2
  [mp4] -> Add8/2
  Gain4/1 -> Add4/1
  [v4] -> Add9/2
  [nq4] -> Add10/2
  Add8/1 -> Add2/4
  Add7/1 -> Add2/5
  Add9/1 -> Add4/4
  Add10/1 -> Add4/5
